simulink model "lab5"  (Simulink 7.1)
settings: Solver=ode45  StartTime=0.0  StopTime=50  RelTol=1e-3
settings Model: Creator=CARLOS BRUNO  LastModifiedBy=CARLOS BRUNO

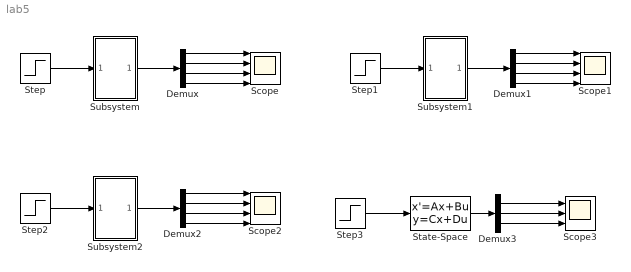
== system lab5 ==
  Demux : Demux
  Demux1 : Demux
  Demux2 : Demux
  Demux3 : Demux  Outputs=3
  Scope : Scope  NumInputPorts=4
      settings: YMin=-5~-5~-5~-5  YMax=5~5~5~5
  Scope1 : Scope  NumInputPorts=4
      settings: YMin=-5~-5~-5~-5  YMax=5~5~5~5
  Scope2 : Scope  NumInputPorts=4
      settings: YMin=-5~-5~-5~-5  YMax=5~5~5~5  SaveName=ScopeData2
  Scope3 : Scope  NumInputPorts=3
      settings: YMin=-5~-5~-5  YMax=5~5~5  SaveName=ScopeData3
  State-Space : StateSpace  A=[-0.25 0.75; -0.25 -0.25]  B=[ 0.5; 0]  C=[-1.5 -1.5 ; 1 0; 0 1]  D=[(3/2); 0; 0]
  Step : Step  Time=0  After=0  SampleTime=0
  Step1 : Step  Time=0  After=0  SampleTime=0
  Step2 : Step  Time=0  Before=1  SampleTime=0
  Step3 : Step  Time=0  Before=1  SampleTime=0
  Subsystem : Subsystem  mask{K=0.5, RC=2}
      mask prompts: K "VARIAVEL K"; RC "VARIAVEL RC"
  Subsystem1 : Subsystem  mask{K=0.5, RC=2}
      mask prompts: K "VARIAVEL K"; RC "VARIAVEL RC"
  Subsystem2 : Subsystem  mask{K=0.5, RC=2}
      mask prompts: K "VARIAVEL K"; RC "VARIAVEL RC"
  wires:
  Step/1 -> Subsystem/1(In1)
  Subsystem/1(Out1) -> Demux/1
  Demux/1 -> Scope/1
  Demux/2 -> Scope/2
  Demux/3 -> Scope/3
  Demux/4 -> Scope/4
  Step1/1 -> Subsystem1/1(In1)
  Subsystem1/1(Out1) -> Demux1/1
  Demux1/1 -> Scope1/1
  Demux1/2 -> Scope1/2
  Demux1/3 -> Scope1/3
  Demux1/4 -> Scope1/4
  Step2/1 -> Subsystem2/1(In1)
  Subsystem2/1(Out1) -> Demux2/1
  Demux2/1 -> Scope2/1
  Demux2/2 -> Scope2/2
  Demux2/3 -> Scope2/3
  Demux2/4 -> Scope2/4
  Demux3/1 -> Scope3/1
  Demux3/2 -> Scope3/2
  Step3/1 -> State-Space/1
  State-Space/1 -> Demux3/1
  Demux3/3 -> Scope3/3

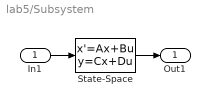
== system lab5/Subsystem ==
  In1 : Inport
  State-Space : StateSpace  A=[-(2 - K)/RC K/RC -(1/RC); K/RC K/RC -(1/RC); (1+2*K)/(2*RC) (1+2*K)/(2*RC) -(1/RC)]  B=[( (2 - K)/RC ); -(K/RC); -(K/RC)]  C=[-(1+K) -(1+K) 0; 1 0 0; 0 1 0; 0 0 1]  D=[(1+K); 0; 0; 0]  X0=[10; 10; 15]
  Out1 : Outport
  wires:
  In1/1 -> State-Space/1
  State-Space/1 -> Out1/1

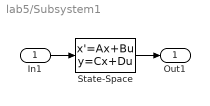
== system lab5/Subsystem1 ==
  In1 : Inport
  State-Space : StateSpace  A=[-(2 - K)/RC K/RC -(1/RC); K/RC K/RC -(1/RC); (1+2*K)/(2*RC) (1+2*K)/(2*RC) -(1/RC)]  B=[( (2 - K)/RC ); -(K/RC); -(K/RC)]  C=[-(1+K) -(1+K) 0; 1 0 0; 0 1 0; 0 0 1]  D=[(1+K); 0; 0; 0]  X0=[10; -10; -10]
  Out1 : Outport
  wires:
  In1/1 -> State-Space/1
  State-Space/1 -> Out1/1

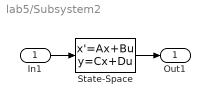
== system lab5/Subsystem2 ==
  In1 : Inport
  State-Space : StateSpace  A=[-(2 - K)/RC K/RC -(1/RC); K/RC K/RC -(1/RC); (1+2*K)/(2*RC) (1+2*K)/(2*RC) -(1/RC)]  B=[( (2 - K)/RC ); -(K/RC); -(K/RC)]  C=[-(1+K) -(1+K) 0; 1 0 0; 0 1 0; 0 0 1]  D=[(1+K); 0; 0; 0]
  Out1 : Outport
  wires:
  In1/1 -> State-Space/1
  State-Space/1 -> Out1/1
